simulink model "hexa_tilted_CAD_FxTESO_ANSFT"  (R2023a)
settings: Solver=ode4  StartTime=0.0  StopTime=60  FixedStep=0.01  RelTol=1e-3
model workspace (MAT data in the model file):
  hover_2m = [0  0  0  0  0  0; 0  0  0  0  0  0; 2  2  2  2  2  2; 0  0  0  0  0  0; 0  0  0  0  0  0; 0  0  0  0  0  0]
  square = [0  0  0  0  0  0; 0  0  0  0  0  0; 2.5  2.5  2.5  2.5  2.5  0; 0  0  0  0  0  0; 0  0  0  0  0  0; 0  0  0  0  0  0]
  tf = Simulink.Parameter
  tf.Value = 60
  tf.DataType = 'auto'
  tf.Complexity = 'real'
  tf.Dimensions = [1 1]
  tray0 = [0  0  0  0  0  0; 0  0  0  0  0  0; 0  5  5  5  5  0; 0  0  0  0  0  0; 0  0  0  0  0  0; 0  0  0  0  0  0]
  tray1 = [0  0  0  0  0  0; 0  0  0  0  0  0; 0  5  2.5  5  2.5  0; 0  0  0  0  0  0; 0  0  0  0  0  0; 0  0  0  0  0  0]
  tray2 = [0  2  2  -2  -2  0; 0  0  -2  -2  2  0; 0  5  2.5  5  2.5  0; 0  0  0  0  0  0; 0  0  0  0  0  0; 0  0  0  0  0  0]
  tray3 = [0  2  2  -2  -2  0; 0  0  -2  -2  2  0; 0  5  2.5  5  2.5  0; 0  0  0  0  0  0; 0  0  0  0  0  0; 0  0  0.785  1.57  0.785  0]
  tray4 = [0  2  2  -2  -2  0; 0  0  -2  -2  2  0; 0  5  2.5  5  2.5  0; 0  0.15  0.15  0.15  0.15  0; 0  0  0  0  0  0; 0  0  0.785  1.57  0.785  0]
  tray5 = [0  0  0  0  0  0; 0  0  0  0  0  0; 0  5  2.5  5  2.5  0; 0  0.15  0.15  0  0  0; 0  0  0.15  0.15  0  0; 0  0  0  0  0  0]
  tray_yaw = [0  0  0  0  0  0; 0  0  0  0  0  0; 0  5  2.5  5  2.5  0; 0  0  0  0  0  0; 0  0  0  0  0  0; 0  0  0.785  1.57  0.785  0]
undefined symbols (not defined in the file or in its folder): F, Light, MIL, smiData, X, Y, Z
libraries: sm_lib x229, nesl_utility x26, sharedtransform x2, robotcorelib x2, mspsensorlib x1, sensorinslib x1, simulink x1, aerolibwind2 x1, SignalEditorBlockLib x1
(part 1 of 6)
settings Model: Creator=adan  LastModifiedBy=adan
settings OptimizationCC: DefaultParameterBehavior=Inlined  EnhancedBackFolding=on  PassReuseOutputArgsAs=Individual arguments  ZeroExternalMemoryAtStartup=off  ZeroInternalMemoryAtStartup=off  OptimizeBlockOrder=speed  DifferentSizesBufferReuse=on  OptimizationCustomize=off  EfficientTunableParamExpr=on
settings DebuggingCC: ParameterTunabilityLossMsg=error
settings SFSimCC: MATLABDynamicMemAlloc=off
settings RTWCC: Description=Embedded Coder  SystemTargetFile=ert.tlc  TemplateMakefile=ert_default_tmf
settings CodeAppCC: ForceParamTrailComments=on  IgnoreCustomStorageClasses=off  OperatorAnnotations=on  SimulinkDataObjDesc=on  SFDataObjDesc=on  InsertBlockDesc=on
settings ERTTargetCC: TargetLangStandard=C99 (ISO)  GenerateSampleERTMain=on  InlinedParameterPlacement=NonHierarchical  ERTCustomFileTemplate=example_file_process.tlc

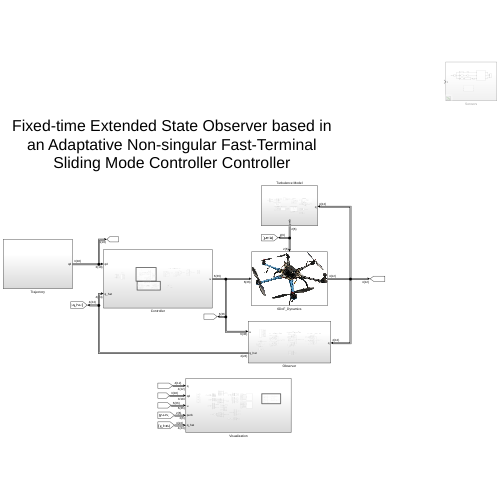
[thumbnail: Simulink's stored preview of the top-level diagram]
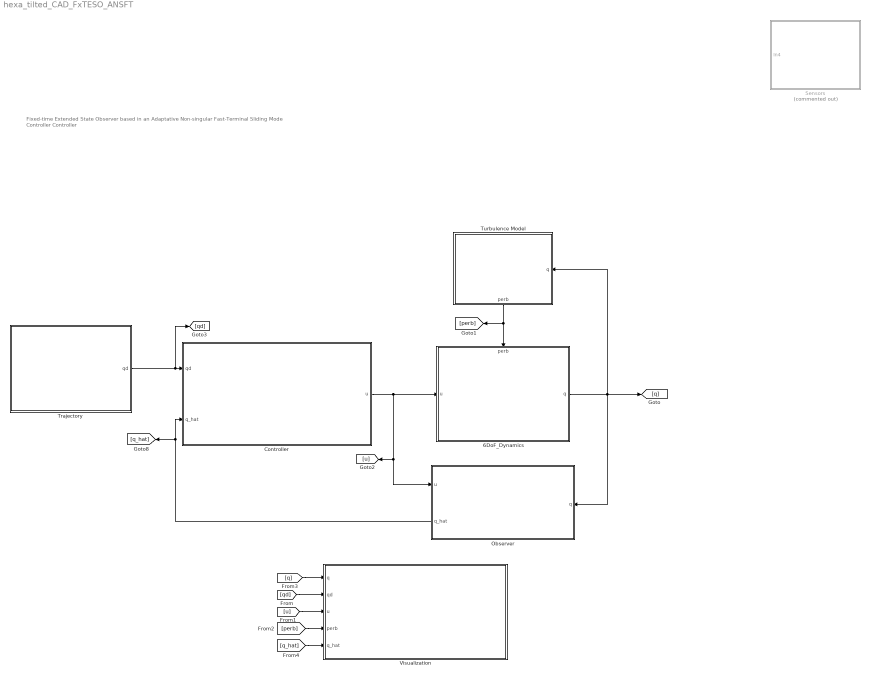
== system hexa_tilted_CAD_FxTESO_ANSFT ==
  note: Fixed-time Extended State Observer based in an Adaptative Non-singular Fast-Terminal Sliding Mode Controller Controller
  6DoF_Dynamics : Subsystem
      settings: PortSchema="{\"entries\":[{\"content\":{\"sides\":[{\"content\":{\"connectorIds\":[\"In1\"]},\"type\":\"ConnectorPlacement.EquallySpacedRectSide\",\"uuid\":\"d79ec49c-5563-41e0-ac59-6e897bc19fda\"},{\"content\":{\"connectorIds\":[\"Out1\"],\"side\":\"RIGHT\"},\"type\":\"ConnectorPlacement.EquallySpacedRectSide\",\"uuid\":\"1255043e-c90e-4bae-9fb4-4fa06f36f53e\"},{\"content\":{\"connectorIds\":[\"In2\"],\"side\":\"TOP\"},\"type\":\"ConnectorPlacement.EquallySpacedRectSide\",\"uuid\":\"823ada36-3f22-4ee3-87a1-180276f622bc\"}]},\"type\":\"ConnectorPlacement.EquallySpacedConnector\",\"uuid\":\"7403b609-b333-4977-a854-ed7a71f74338\"}],\"packageUris\":[\"http://schema.mathworks.com/mf0/Connector/R2020b\"],\"version\":\"1.0\"}"
      mask Display: image('/home/adan/Descargas/hexatilted.jpeg'); % Use "Edit Image" on toolstrip to change.
  Controller : Subsystem
  Observer : Subsystem
      settings: PortSchema="{\"entries\":[{\"content\":{\"sides\":[{\"content\":{\"connectorIds\":[\"In1\",\"Out1\"]},\"type\":\"ConnectorPlacement.EquallySpacedRectSide\",\"uuid\":\"d79ec49c-5563-41e0-ac59-6e897bc19fda\"},{\"content\":{\"connectorIds\":[\"In2\"],\"side\":\"RIGHT\"},\"type\":\"ConnectorPlacement.EquallySpacedRectSide\",\"uuid\":\"1255043e-c90e-4bae-9fb4-4fa06f36f53e\"},{\"content\":{\"side\":\"TOP\"},\"type\":\"ConnectorPlacement.EquallySpacedRectSide\",\"uuid\":\"823ada36-3f22-4ee3-87a1-180276f622bc\"}]},\"type\":\"ConnectorPlacement.EquallySpacedConnector\",\"uuid\":\"7403b609-b333-4977-a854-ed7a71f74338\"}],\"packageUris\":[\"http://schema.mathworks.com/mf0/Connector/R2020b\"],\"version\":\"1.0\"}"
  Sensors : Subsystem  Commented=on
  Trajectory : Subsystem
  Turbulence Model : Subsystem
      settings: PortSchema="{\"entries\":[{\"content\":{\"sides\":[{\"content\":{},\"type\":\"ConnectorPlacement.EquallySpacedRectSide\",\"uuid\":\"1a11629b-61d3-4a8e-8df8-8509e014e579\"},{\"content\":{\"connectorIds\":[\"In1\"],\"side\":\"RIGHT\"},\"type\":\"ConnectorPlacement.EquallySpacedRectSide\",\"uuid\":\"4b15c564-9714-4da5-9436-a08c0d95800f\"},{\"content\":{\"side\":\"TOP\"},\"type\":\"ConnectorPlacement.EquallySpacedRectSide\",\"uuid\":\"dd21b825-2def-4360-b27b-b8c6f475bfab\"},{\"content\":{\"connectorIds\":[\"Out1\"],\"side\":\"BOTTOM\"},\"type\":\"ConnectorPlacement.EquallySpacedRectSide\",\"uuid\":\"06c31a07-f778-4273-8a03-7a766e1c2883\"}]},\"type\":\"ConnectorPlacement.EquallySpacedConnector\",\"uuid\":\"4c6e67eb-825c-4dd0-a48b-2afa68ae74f5\"}],\"packageUris\":[\"http://schema.mathworks.com/mf0/Connector/R2020b\"],\"version\":\"1.0\"}"
  Visualization : Subsystem
  wires:
  Trajectory/1(qd) -> [qd], Controller/1(qd)
  Controller/1(u) -> 6DoF_Dynamics/1(u), [u], Observer/1(u)
  6DoF_Dynamics/1(q) -> Turbulence Model/1(q), [q], Observer/2(q)
  Observer/1(q_hat) -> [q_hat], Controller/2(q_hat)
  [qd] -> Visualization/2(qd)
  [u] -> Visualization/3(u)
  [perb] -> Visualization/4(perb)
  [q_hat] -> Visualization/5(q_hat)
  [q] -> Visualization/1(q)
  Turbulence Model/1(perb) -> 6DoF_Dynamics/2(perb), [perb]

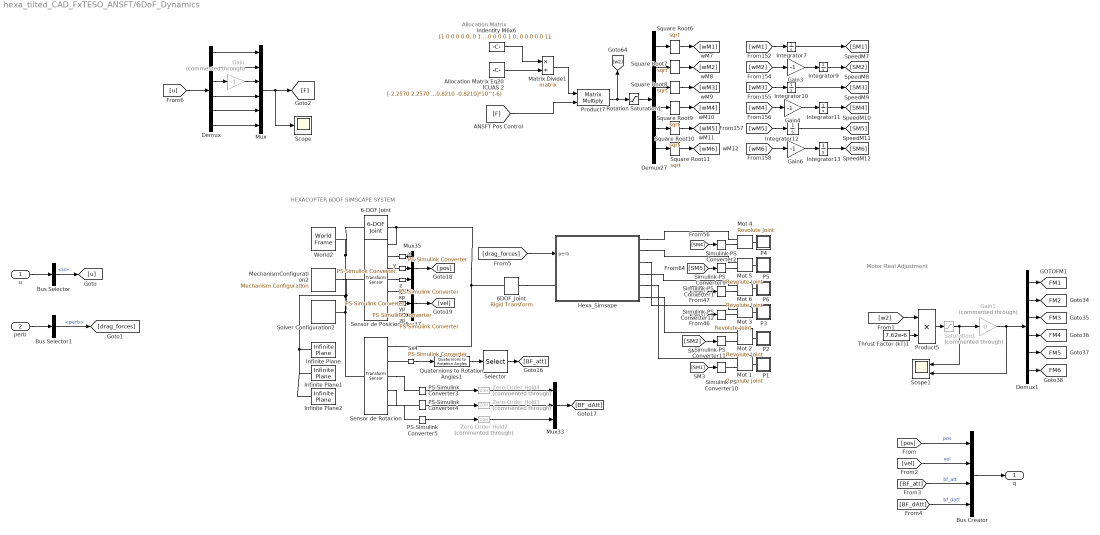
== system hexa_tilted_CAD_FxTESO_ANSFT/6DoF_Dynamics ==
  note: Motor Real Adjustment
  note: Allocation Matrix
  note: HEXACOPTER 6DOF SIMSCAPE SYSTEM
  u : Inport
  perb : Inport  Port=2
  6-DOF Joint : sm_lib/Joints/6-DOF Joint  JointMode=Normal  SenseConstraintForce=off  SenseConstraintForceX=off  SenseConstraintForceY=off  SenseConstraintForceZ=off  SenseConstraintTorque=off  SenseConstraintTorqueX=off  SenseConstraintTorqueY=off  SenseConstraintTorqueZ=off  SenseTotalForce=off  SenseTotalForceX=off  SenseTotalForceY=off  SenseTotalForceZ=off  SenseTotalTorque=off  SenseTotalTorqueX=off  SenseTotalTorqueY=off  SenseTotalTorqueZ=off  CompositeWrenchDir=FollowerOnBase  CompositeWrenchFrame=BaseFrame  PxEquilibriumPosition=0  PxEquilibriumPositionUnits=m  PxSpringStiffness=0  PxSpringStiffnessUnits=N/m  PxDampingCoefficient=0  PxDampingCoefficientUnits=N/(m/s)  PxTorqueActuationMode=NoTorque  PxMotionActuationMode=ComputedMotion  PxSensePosition=off  PxSenseVelocity=off  PxSenseAcceleration=off  PxSenseTorqueForce=off  PxSenseLowerLimitTorqueForce=off  PxSenseUpperLimitTorqueForce=off  PxLowerLimitSpecify=off  PxLowerLimitBound=-1  PxLowerLimitBoundUnits=m  PxLowerLimitStiffness=1e6  PxLowerLimitStiffnessUnits=N/m  PxLowerLimitDamping=1e3  PxLowerLimitDampingUnits=N/(m/s)  PxLowerLimitTransitionRegionWidth=1e-4  PxLowerLimitTransitionRegionWidthUnits=m  PxUpperLimitSpecify=off  PxUpperLimitBound=1  PxUpperLimitBoundUnits=m  PxUpperLimitStiffness=1e6  PxUpperLimitStiffnessUnits=N/m  PxUpperLimitDamping=1e3  PxUpperLimitDampingUnits=N/(m/s)  PxUpperLimitTransitionRegionWidth=1e-4  PxUpperLimitTransitionRegionWidthUnits=m  PxPositionTargetSpecify=off  PxPositionTargetPriority=High  PxPositionTargetValue=0  PxPositionTargetValueUnits=m  PxVelocityTargetSpecify=off  PxVelocityTargetPriority=High  PxVelocityTargetValue=0  PxVelocityTargetValueUnits=m/s  PyEquilibriumPosition=0  PyEquilibriumPositionUnits=m  PySpringStiffness=0  PySpringStiffnessUnits=N/m  PyDampingCoefficient=0  PyDampingCoefficientUnits=N/(m/s)  PyTorqueActuationMode=NoTorque  PyMotionActuationMode=ComputedMotion  PySensePosition=off  PySenseVelocity=off  PySenseAcceleration=off  PySenseTorqueForce=off  PySenseLowerLimitTorqueForce=off  PySenseUpperLimitTorqueForce=off  PyLowerLimitSpecify=off  PyLowerLimitBound=-1  PyLowerLimitBoundUnits=m  PyLowerLimitStiffness=1e6  PyLowerLimitStiffnessUnits=N/m  PyLowerLimitDamping=1e3  PyLowerLimitDampingUnits=N/(m/s)  PyLowerLimitTransitionRegionWidth=1e-4  PyLowerLimitTransitionRegionWidthUnits=m  PyUpperLimitSpecify=off  PyUpperLimitBound=1  PyUpperLimitBoundUnits=m  PyUpperLimitStiffness=1e6  PyUpperLimitStiffnessUnits=N/m  PyUpperLimitDamping=1e3  PyUpperLimitDampingUnits=N/(m/s)  PyUpperLimitTransitionRegionWidth=1e-4  PyUpperLimitTransitionRegionWidthUnits=m  PyPositionTargetSpecify=off  PyPositionTargetPriority=High  PyPositionTargetValue=0  PyPositionTargetValueUnits=m  PyVelocityTargetSpecify=off  PyVelocityTargetPriority=High  PyVelocityTargetValue=0  PyVelocityTargetValueUnits=m/s  PzEquilibriumPosition=0  PzEquilibriumPositionUnits=m  PzSpringStiffness=0  PzSpringStiffnessUnits=N/m  PzDampingCoefficient=0  PzDampingCoefficientUnits=N/(m/s)  PzTorqueActuationMode=NoTorque  PzMotionActuationMode=ComputedMotion  PzSensePosition=off  PzSenseVelocity=off  PzSenseAcceleration=off  PzSenseTorqueForce=off  PzSenseLowerLimitTorqueForce=off  PzSenseUpperLimitTorqueForce=off  PzLowerLimitSpecify=off  PzLowerLimitBound=-1  PzLowerLimitBoundUnits=m  PzLowerLimitStiffness=1e6  PzLowerLimitStiffnessUnits=N/m  PzLowerLimitDamping=1e3  PzLowerLimitDampingUnits=N/(m/s)  PzLowerLimitTransitionRegionWidth=1e-4  PzLowerLimitTransitionRegionWidthUnits=m  PzUpperLimitSpecify=off  PzUpperLimitBound=1  PzUpperLimitBoundUnits=m  PzUpperLimitStiffness=1e6  PzUpperLimitStiffnessUnits=N/m  PzUpperLimitDamping=1e3  PzUpperLimitDampingUnits=N/(m/s)  PzUpperLimitTransitionRegionWidth=1e-4  PzUpperLimitTransitionRegionWidthUnits=m  PzPositionTargetSpecify=on  PzPositionTargetPriority=High  PzPositionTargetValue=0.20  PzPositionTargetValueUnits=m  PzVelocityTargetSpecify=off  PzVelocityTargetPriority=High  PzVelocityTargetValue=0  PzVelocityTargetValueUnits=m/s  SphEqPosRotationMethod=None  SphEqPosRotationAngleUnits=deg  SphEqPosRotationStandardAxis=+Z  SphEqPosRotationAngle=0.0  SphEqPosRotationArbitraryAxis=[0 0 1]  SphEqPosFollAlignAxisA=+X  SphEqPosBaseAlignAxisA=+Y  SphEqPosFollAlignAxisB=+Y  SphEqPosBaseAlignAxisB=+Z  SphEqPosRotationSequenceAxes=FollowerAxes  SphEqPosRotationSequence=XYX  SphEqPosRotationSequenceAngles=[0 0 0]  SphEqPosRotationSequenceAnglesUnits=deg  SphEqPosRotationMatrix=[1 0 0; 0 1 0; 0 0 1]  SphEqPosQuaternion=[1 0 0 0]  SphSpringStiffness=0  SphSpringStiffnessUnits=N*m/deg  SphDampingCoefficient=0  SphDampingCoefficientUnits=N*m/(deg/s)  SphActuateTorqueX=off  SphActuateTorqueY=off  SphActuateTorqueZ=off  SphActuateTorque=off  SphTorqueActuationMode=NoTorque  SphMotionActuationMode=ComputedMotion  SphActuationFrame=BaseFrame  SphSensePosition=off  SphSenseVelocityX=off  SphSenseVelocityY=off  SphSenseVelocityZ=off  SphSenseVelocity=off  SphSenseAccelerationX=off  SphSenseAccelerationY=off  SphSenseAccelerationZ=off  SphSenseAcceleration=off  SphSenseTorqueX=off  SphSenseTorqueY=off  SphSenseTorqueZ=off  SphSenseTorqueForce=off  SphSenseLowerLimitTorqueMag=off  SphSenseUpperLimitTorqueMag=off  SphSensingFrame=BaseFrame  SphLowerLimitSpecify=off  SphLowerLimitBound=15  SphLowerLimitBoundUnits=deg  SphLowerLimitStiffness=1e4  SphLowerLimitStiffnessUnits=N*m/deg  SphLowerLimitDamping=10  SphLowerLimitDampingUnits=N*m/(deg/s)  SphLowerLimitTransitionRegionWidth=0.1  SphLowerLimitTransitionRegionWidthUnits=deg  SphUpperLimitSpecify=off  SphUpperLimitBound=45  SphUpperLimitBoundUnits=deg  SphUpperLimitStiffness=1e4  SphUpperLimitStiffnessUnits=N*m/deg  SphUpperLimitDamping=10  SphUpperLimitDampingUnits=N*m/(deg/s)  SphUpperLimitTransitionRegionWidth=0.1  SphUpperLimitTransitionRegionWidthUnits=deg  SphPositionTargetRotationMethod=StandardAxis  SphPositionTargetRotationAngleUnits=deg  SphPositionTargetRotationStandardAxis=+Z  SphPositionTargetRotationAngle=-45  SphPositionTargetRotationArbitraryAxis=[0 0 1]  SphPositionTargetFollAlignAxisA=+X  SphPositionTargetBaseAlignAxisA=+Y  SphPositionTargetFollAlignAxisB=+Y  SphPositionTargetBaseAlignAxisB=+Z  SphPositionTargetRotationSequenceAxes=FollowerAxes  SphPositionTargetRotationSequence=XYX  SphPositionTargetRotationSequenceAngles=[0 0 0]  SphPositionTargetRotationSequenceAnglesUnits=deg  SphPositionTargetRotationMatrix=[1 0 0; 0 1 0; 0 0 1]  SphPositionTargetQuaternion=[1 0 0 0]  SphPositionTargetSpecify=off  SphPositionTargetPriority=High  SphVelocityTargetValue=[0 0 0]  SphVelocityTargetValueUnits=deg/s  SphVelocityTargetSpecify=off  SphVelocityTargetPriority=High  SphVelocityTargetInFollowerFrame=on
  6DOF_Joint : sm_lib/Frames and Transforms/Rigid Transform  TranslationMethod=Cartesian  TranslationStandardOffset=-0.185  TranslationStandardOffsetUnits=m  TranslationStandardAxis=+Z  TranslationCartesianOffset=[0.0195 0.01 -0.26]  TranslationCartesianOffsetUnits=m  TranslationROffset=0  TranslationROffsetUnits=m  TranslationZOffset=0  TranslationZOffsetUnits=m  TranslationThetaOffset=0  TranslationThetaOffsetUnits=deg  RotationMethod=RotationMatrix  RotationAngleUnits=deg  RotationStandardAxis=+Z  RotationAngle=0.0  RotationArbitraryAxis=[0 0 1]  FollAlignAxisA=+X  BaseAlignAxisA=+Y  FollAlignAxisB=+Y  BaseAlignAxisB=+Z  RotationSequenceAxes=FollowerAxes  RotationSequence=XYX  RotationSequenceAngles=[0 0 0]  RotationSequenceAnglesUnits=deg  RotationMatrix=[1 0 0; 0 1 0; 0 0 1]  Quaternion=[1 0 0 0]
  Allocation Matrix Eq20 ICUAS 2 : Constant  Value=[-2.2570 2.2570 0 -2.2570 2.2570 0; 1.3030 1.3030 -2.6060 1.3030 1.3030 -2.6060; 7.160 7.160 7.160 7.160 7.160 7.160; 1.6370 1.6370 0 -1.6370 -1.6370 0; -0.945 0.945 1.891 0.945 -0.945 -1.891; 0.8210 -0.8210 0.8210 -0.8210 0.8210 -0.8210]*10^(-6)
  Bus Creator : BusCreator  Inputs=4
  Bus Selector : BusSelector  OutputSignals=u
  Bus Selector1 : BusSelector  OutputSignals=perb
  Demux : Demux  Outputs=6
  Demux1 : Demux  Outputs=6
  Demux27 : Demux  Outputs=6
  Gain : Gain  Commented=through  Gain=-1
  Gain1 : Gain  Commented=through  Gain=0
  Gain3 : Gain  Gain=-1
  Gain4 : Gain  Gain=-1
  Gain6 : Gain  Gain=-1
  Hexa_Simsape : Subsystem
      mask Display: image('$imagefile'); % Use "Edit Image" on toolstrip to change.
  Indentity M6x6 : Constant  Value=[1 0 0 0 0 0; 0 1 0 0 0 0; 0 0 1 0 0 0; 0 0 0 1 0 0; 0 0 0 0 1 0; 0 0 0 0 0 1];
  Infinite Plane : sm_lib/Curves and Surfaces/Infinite Plane  GraphicType=Rectangle  GraphicPlaneWidth=8  GraphicPlaneWidthUnits=m  GraphicPlaneHeight=5  GraphicPlaneHeightUnits=m  GraphicVisPropType=SimpleVisualProperties  GraphicDiffuseColor=[1 1 0.06667]  GraphicOpacity=0.25  GraphicSpecularColor=[1 1 1]  GraphicAmbientColor=[1 1 1]  GraphicEmissiveColor=[1 1 1]  GraphicShininess=75
  Infinite Plane1 : sm_lib/Curves and Surfaces/Infinite Plane  GraphicType=Rectangle  GraphicPlaneWidth=8  GraphicPlaneWidthUnits=m  GraphicPlaneHeight=0.01  GraphicPlaneHeightUnits=m  GraphicVisPropType=SimpleVisualProperties  GraphicDiffuseColor=[1 1 0.06667]  GraphicOpacity=0.5  GraphicSpecularColor=[0.5 0.5 0.5 1.0]  GraphicAmbientColor=[0.15 0.15 0.15 1.0]  GraphicEmissiveColor=[0.0 0.0 0.0 1.0]  GraphicShininess=75
  Infinite Plane2 : sm_lib/Curves and Surfaces/Infinite Plane  GraphicType=Rectangle  GraphicPlaneWidth=0.01  GraphicPlaneWidthUnits=m  GraphicPlaneHeight=5  GraphicPlaneHeightUnits=m  GraphicVisPropType=SimpleVisualProperties  GraphicDiffuseColor=[1 1 0.06667]  GraphicOpacity=0.5  GraphicSpecularColor=[0.5 0.5 0.5 1.0]  GraphicAmbientColor=[0.15 0.15 0.15 1.0]  GraphicEmissiveColor=[0.0 0.0 0.0 1.0]  GraphicShininess=75
  Integrator{7,9..13} (6 alike) : Integrator
  Matrix Divide1 : Product  Inputs=*/  Multiplication=Matrix(*)
  MechanismConfiguration2 : sm_lib/Utilities/Mechanism Configuration  UniformGravity=Constant  GravityVector=[0 0 -9.80665]  GravityVectorUnits=m/s^2  LinearizationDelta=0.01  JointModeTransitionNonlinearIterations=2
  Mot 1 : sm_lib/Joints/Revolute Joint  JointMode=Normal  SenseConstraintForce=off  SenseConstraintForceX=off  SenseConstraintForceY=off  SenseConstraintForceZ=off  SenseConstraintTorque=off  SenseConstraintTorqueX=off  SenseConstraintTorqueY=off  SenseConstraintTorqueZ=off  SenseTotalForce=off  SenseTotalForceX=off  SenseTotalForceY=off  SenseTotalForceZ=off  SenseTotalTorque=off  SenseTotalTorqueX=off  SenseTotalTorqueY=off  SenseTotalTorqueZ=off  CompositeWrenchDir=FollowerOnBase  CompositeWrenchFrame=BaseFrame  EquilibriumPosition=0  EquilibriumPositionUnits=deg  SpringStiffness=0  SpringStiffnessUnits=N*m/deg  DampingCoefficient=0  DampingCoefficientUnits=N*m/(deg/s)  TorqueActuationMode=ComputedTorque  MotionActuationMode=InputMotion  SensePosition=off  SenseVelocity=off  SenseAcceleration=off  SenseTorqueForce=off  SenseLowerLimitTorqueForce=off  SenseUpperLimitTorqueForce=off  LowerLimitSpecify=off  LowerLimitBound=-90  LowerLimitBoundUnits=deg  LowerLimitStiffness=1e4  LowerLimitStiffnessUnits=N*m/deg  LowerLimitDamping=10  LowerLimitDampingUnits=N*m/(deg/s)  LowerLimitTransitionRegionWidth=0.1  LowerLimitTransitionRegionWidthUnits=deg  UpperLimitSpecify=off  UpperLimitBound=90  UpperLimitBoundUnits=deg  UpperLimitStiffness=1e4  UpperLimitStiffnessUnits=N*m/deg  UpperLimitDamping=10  UpperLimitDampingUnits=N*m/(deg/s)  UpperLimitTransitionRegionWidth=0.1  UpperLimitTransitionRegionWidthUnits=deg  PositionTargetSpecify=on  PositionTargetPriority=Low  PositionTargetValue=smiData.RevoluteJoint(1).Rz.Pos  PositionTargetValueUnits=deg  VelocityTargetSpecify=off  VelocityTargetPriority=High  VelocityTargetValue=0  VelocityTargetValueUnits=deg/s
  Mot 2 : sm_lib/Joints/Revolute Joint  JointMode=Normal  SenseConstraintForce=off  SenseConstraintForceX=off  SenseConstraintForceY=off  SenseConstraintForceZ=off  SenseConstraintTorque=off  SenseConstraintTorqueX=off  SenseConstraintTorqueY=off  SenseConstraintTorqueZ=off  SenseTotalForce=off  SenseTotalForceX=off  SenseTotalForceY=off  SenseTotalForceZ=off  SenseTotalTorque=off  SenseTotalTorqueX=off  SenseTotalTorqueY=off  SenseTotalTorqueZ=off  CompositeWrenchDir=FollowerOnBase  CompositeWrenchFrame=BaseFrame  EquilibriumPosition=0  EquilibriumPositionUnits=deg  SpringStiffness=0  SpringStiffnessUnits=N*m/deg  DampingCoefficient=0  DampingCoefficientUnits=N*m/(deg/s)  TorqueActuationMode=ComputedTorque  MotionActuationMode=InputMotion  SensePosition=off  SenseVelocity=off  SenseAcceleration=off  SenseTorqueForce=off  SenseLowerLimitTorqueForce=off  SenseUpperLimitTorqueForce=off  LowerLimitSpecify=off  LowerLimitBound=-90  LowerLimitBoundUnits=deg  LowerLimitStiffness=1e4  LowerLimitStiffnessUnits=N*m/deg  LowerLimitDamping=10  LowerLimitDampingUnits=N*m/(deg/s)  LowerLimitTransitionRegionWidth=0.1  LowerLimitTransitionRegionWidthUnits=deg  UpperLimitSpecify=off  UpperLimitBound=90  UpperLimitBoundUnits=deg  UpperLimitStiffness=1e4  UpperLimitStiffnessUnits=N*m/deg  UpperLimitDamping=10  UpperLimitDampingUnits=N*m/(deg/s)  UpperLimitTransitionRegionWidth=0.1  UpperLimitTransitionRegionWidthUnits=deg  PositionTargetSpecify=on  PositionTargetPriority=Low  PositionTargetValue=smiData.RevoluteJoint(2).Rz.Pos  PositionTargetValueUnits=deg  VelocityTargetSpecify=off  VelocityTargetPriority=High  VelocityTargetValue=0  VelocityTargetValueUnits=deg/s
  Mot 3 : sm_lib/Joints/Revolute Joint  JointMode=Normal  SenseConstraintForce=off  SenseConstraintForceX=off  SenseConstraintForceY=off  SenseConstraintForceZ=off  SenseConstraintTorque=off  SenseConstraintTorqueX=off  SenseConstraintTorqueY=off  SenseConstraintTorqueZ=off  SenseTotalForce=off  SenseTotalForceX=off  SenseTotalForceY=off  SenseTotalForceZ=off  SenseTotalTorque=off  SenseTotalTorqueX=off  SenseTotalTorqueY=off  SenseTotalTorqueZ=off  CompositeWrenchDir=FollowerOnBase  CompositeWrenchFrame=BaseFrame  EquilibriumPosition=0  EquilibriumPositionUnits=deg  SpringStiffness=0  SpringStiffnessUnits=N*m/deg  DampingCoefficient=0  DampingCoefficientUnits=N*m/(deg/s)  TorqueActuationMode=ComputedTorque  MotionActuationMode=InputMotion  SensePosition=off  SenseVelocity=off  SenseAcceleration=off  SenseTorqueForce=off  SenseLowerLimitTorqueForce=off  SenseUpperLimitTorqueForce=off  LowerLimitSpecify=off  LowerLimitBound=-90  LowerLimitBoundUnits=deg  LowerLimitStiffness=1e4  LowerLimitStiffnessUnits=N*m/deg  LowerLimitDamping=10  LowerLimitDampingUnits=N*m/(deg/s)  LowerLimitTransitionRegionWidth=0.1  LowerLimitTransitionRegionWidthUnits=deg  UpperLimitSpecify=off  UpperLimitBound=90  UpperLimitBoundUnits=deg  UpperLimitStiffness=1e4  UpperLimitStiffnessUnits=N*m/deg  UpperLimitDamping=10  UpperLimitDampingUnits=N*m/(deg/s)  UpperLimitTransitionRegionWidth=0.1  UpperLimitTransitionRegionWidthUnits=deg  PositionTargetSpecify=on  PositionTargetPriority=Low  PositionTargetValue=smiData.RevoluteJoint(3).Rz.Pos  PositionTargetValueUnits=deg  VelocityTargetSpecify=off  VelocityTargetPriority=High  VelocityTargetValue=0  VelocityTargetValueUnits=deg/s
  Mot 4 : sm_lib/Joints/Revolute Joint  JointMode=Normal  SenseConstraintForce=off  SenseConstraintForceX=off  SenseConstraintForceY=off  SenseConstraintForceZ=off  SenseConstraintTorque=off  SenseConstraintTorqueX=off  SenseConstraintTorqueY=off  SenseConstraintTorqueZ=off  SenseTotalForce=off  SenseTotalForceX=off  SenseTotalForceY=off  SenseTotalForceZ=off  SenseTotalTorque=off  SenseTotalTorqueX=off  SenseTotalTorqueY=off  SenseTotalTorqueZ=off  CompositeWrenchDir=FollowerOnBase  CompositeWrenchFrame=BaseFrame  EquilibriumPosition=0  EquilibriumPositionUnits=deg  SpringStiffness=0  SpringStiffnessUnits=N*m/deg  DampingCoefficient=0  DampingCoefficientUnits=N*m/(deg/s)  TorqueActuationMode=ComputedTorque  MotionActuationMode=InputMotion  SensePosition=off  SenseVelocity=off  SenseAcceleration=off  SenseTorqueForce=off  SenseLowerLimitTorqueForce=off  SenseUpperLimitTorqueForce=off  LowerLimitSpecify=off  LowerLimitBound=-90  LowerLimitBoundUnits=deg  LowerLimitStiffness=1e4  LowerLimitStiffnessUnits=N*m/deg  LowerLimitDamping=10  LowerLimitDampingUnits=N*m/(deg/s)  LowerLimitTransitionRegionWidth=0.1  LowerLimitTransitionRegionWidthUnits=deg  UpperLimitSpecify=off  UpperLimitBound=90  UpperLimitBoundUnits=deg  UpperLimitStiffness=1e4  UpperLimitStiffnessUnits=N*m/deg  UpperLimitDamping=10  UpperLimitDampingUnits=N*m/(deg/s)  UpperLimitTransitionRegionWidth=0.1  UpperLimitTransitionRegionWidthUnits=deg  PositionTargetSpecify=on  PositionTargetPriority=Low  PositionTargetValue=smiData.RevoluteJoint(5).Rz.Pos  PositionTargetValueUnits=deg  VelocityTargetSpecify=off  VelocityTargetPriority=High  VelocityTargetValue=0  VelocityTargetValueUnits=deg/s
  Mot 5 : sm_lib/Joints/Revolute Joint  JointMode=Normal  SenseConstraintForce=off  SenseConstraintForceX=off  SenseConstraintForceY=off  SenseConstraintForceZ=off  SenseConstraintTorque=off  SenseConstraintTorqueX=off  SenseConstraintTorqueY=off  SenseConstraintTorqueZ=off  SenseTotalForce=off  SenseTotalForceX=off  SenseTotalForceY=off  SenseTotalForceZ=off  SenseTotalTorque=off  SenseTotalTorqueX=off  SenseTotalTorqueY=off  SenseTotalTorqueZ=off  CompositeWrenchDir=FollowerOnBase  CompositeWrenchFrame=BaseFrame  EquilibriumPosition=0  EquilibriumPositionUnits=deg  SpringStiffness=0  SpringStiffnessUnits=N*m/deg  DampingCoefficient=0  DampingCoefficientUnits=N*m/(deg/s)  TorqueActuationMode=ComputedTorque  MotionActuationMode=InputMotion  SensePosition=off  SenseVelocity=off  SenseAcceleration=off  SenseTorqueForce=off  SenseLowerLimitTorqueForce=off  SenseUpperLimitTorqueForce=off  LowerLimitSpecify=off  LowerLimitBound=-90  LowerLimitBoundUnits=deg  LowerLimitStiffness=1e4  LowerLimitStiffnessUnits=N*m/deg  LowerLimitDamping=10  LowerLimitDampingUnits=N*m/(deg/s)  LowerLimitTransitionRegionWidth=0.1  LowerLimitTransitionRegionWidthUnits=deg  UpperLimitSpecify=off  UpperLimitBound=90  UpperLimitBoundUnits=deg  UpperLimitStiffness=1e4  UpperLimitStiffnessUnits=N*m/deg  UpperLimitDamping=10  UpperLimitDampingUnits=N*m/(deg/s)  UpperLimitTransitionRegionWidth=0.1  UpperLimitTransitionRegionWidthUnits=deg  PositionTargetSpecify=on  PositionTargetPriority=Low  PositionTargetValue=smiData.RevoluteJoint(6).Rz.Pos  PositionTargetValueUnits=deg  VelocityTargetSpecify=off  VelocityTargetPriority=High  VelocityTargetValue=0  VelocityTargetValueUnits=deg/s
  Mot 6 : sm_lib/Joints/Revolute Joint  JointMode=Normal  SenseConstraintForce=off  SenseConstraintForceX=off  SenseConstraintForceY=off  SenseConstraintForceZ=off  SenseConstraintTorque=off  SenseConstraintTorqueX=off  SenseConstraintTorqueY=off  SenseConstraintTorqueZ=off  SenseTotalForce=off  SenseTotalForceX=off  SenseTotalForceY=off  SenseTotalForceZ=off  SenseTotalTorque=off  SenseTotalTorqueX=off  SenseTotalTorqueY=off  SenseTotalTorqueZ=off  CompositeWrenchDir=FollowerOnBase  CompositeWrenchFrame=BaseFrame  EquilibriumPosition=0  EquilibriumPositionUnits=deg  SpringStiffness=0  SpringStiffnessUnits=N*m/deg  DampingCoefficient=0  DampingCoefficientUnits=N*m/(deg/s)  TorqueActuationMode=ComputedTorque  MotionActuationMode=InputMotion  SensePosition=off  SenseVelocity=off  SenseAcceleration=off  SenseTorqueForce=off  SenseLowerLimitTorqueForce=off  SenseUpperLimitTorqueForce=off  LowerLimitSpecify=off  LowerLimitBound=-90  LowerLimitBoundUnits=deg  LowerLimitStiffness=1e4  LowerLimitStiffnessUnits=N*m/deg  LowerLimitDamping=10  LowerLimitDampingUnits=N*m/(deg/s)  LowerLimitTransitionRegionWidth=0.1  LowerLimitTransitionRegionWidthUnits=deg  UpperLimitSpecify=off  UpperLimitBound=90  UpperLimitBoundUnits=deg  UpperLimitStiffness=1e4  UpperLimitStiffnessUnits=N*m/deg  UpperLimitDamping=10  UpperLimitDampingUnits=N*m/(deg/s)  UpperLimitTransitionRegionWidth=0.1  UpperLimitTransitionRegionWidthUnits=deg  PositionTargetSpecify=on  PositionTargetPriority=Low  PositionTargetValue=smiData.RevoluteJoint(4).Rz.Pos  PositionTargetValueUnits=deg  VelocityTargetSpecify=off  VelocityTargetPriority=High  VelocityTargetValue=0  VelocityTargetValueUnits=deg/s
  Mux : Mux  Inputs=6
  Mux33 : Mux  Inputs=3
  Mux35 : Mux  Inputs=3
  Mux37 : Mux  Inputs=3
  P1 : Subsystem
  P2 : Subsystem
  P3 : Subsystem
  P4 : Subsystem
  P5 : Subsystem
  P6 : Subsystem
  PS-Simulink Converter3 : nesl_utility/PS-Simulink Converter  PhysicalDomain=network_engine_domain  SubClassName=ps_output  LeftPortType=input  RightPortType=output  PseudoPeriodic=off  Frequencies=[]  VectorFormat=1-D array  Unit=inherit  AffineConversion=off
  PS-Simulink Converter4 : nesl_utility/PS-Simulink Converter  PhysicalDomain=network_engine_domain  SubClassName=ps_output  LeftPortType=input  RightPortType=output  PseudoPeriodic=off  Frequencies=[]  VectorFormat=1-D array  Unit=inherit  AffineConversion=off
  PS-Simulink Converter5 : nesl_utility/PS-Simulink Converter  PhysicalDomain=network_engine_domain  SubClassName=ps_output  LeftPortType=input  RightPortType=output  PseudoPeriodic=off  Frequencies=[]  VectorFormat=1-D array  Unit=inherit  AffineConversion=off
  Product5 : Product
  Product7 : Product  Multiplication=Matrix(*)
  Quaternions to Rotation Angles1 : sharedtransform/Quaternions to Rotation Angles  rotationOrder=ZYX  aMode=aMode
  Rotation Saturation1 : Saturate  UpperLimit=1.4e6  LowerLimit=0
  Saturation1 : Saturate  Commented=through  UpperLimit=10  LowerLimit=0
  Scope : Scope
  Scope1 : Scope  NumInputPorts=2
  Selector : Selector  InputPortWidth=3  IndexOptions=Index vector (dialog)  Indices=[3 2 1]  OutputSizes=1
  Sensor de Posicion : sm_lib/Frames and Transforms/Transform Sensor  MeasurementFrame=World  RotationSequence=XYX  SenseAngle=off  SenseAxis=off  SenseQ=off  SenseR=off  SenseRotationSequence=off  SenseOmegaX=off  SenseOmegaY=off  SenseOmegaZ=off  SenseQDot=off  SenseRDot=off  SenseRotationSequenceDot=off  SenseAlphaX=off  SenseAlphaY=off  SenseAlphaZ=off  SenseQDDot=off  SenseRDDot=off  SenseX=on  SenseY=on  SenseZ=on  SenseRad=off  SenseAzim=off  SenseDist=off  SenseInc=off  SenseXDot=on  SenseYDot=on  SenseZDot=on  SenseRadDot=off  SenseAzimDot=off  SenseDistDot=off  SenseIncDot=off  SenseXDDot=off  SenseYDDot=off  SenseZDDot=off  SenseRadDDot=off  SenseAzimDDot=off  SenseDistDDot=off  SenseIncDDot=off
  Sensor de Rotacion : sm_lib/Frames and Transforms/Transform Sensor  MeasurementFrame=Follower  RotationSequence=XYX  SenseAngle=off  SenseAxis=off  SenseQ=on  SenseR=off  SenseRotationSequence=off  SenseOmegaX=on  SenseOmegaY=on  SenseOmegaZ=on  SenseQDot=off  SenseRDot=off  SenseRotationSequenceDot=off  SenseAlphaX=off  SenseAlphaY=off  SenseAlphaZ=off  SenseQDDot=off  SenseRDDot=off  SenseX=off  SenseY=off  SenseZ=off  SenseRad=off  SenseAzim=off  SenseDist=off  SenseInc=off  SenseXDot=off  SenseYDot=off  SenseZDot=off  SenseRadDot=off  SenseAzimDot=off  SenseDistDot=off  SenseIncDot=off  SenseXDDot=off  SenseYDDot=off  SenseZDDot=off  SenseRadDDot=off  SenseAzimDDot=off  SenseDistDDot=off  SenseIncDDot=off
  Simulink-PS Converter{1..2,9..12} (6 alike) : nesl_utility/Simulink-PS Converter  PhysicalDomain=network_engine_domain  SubClassName=ps_input  LeftPortType=input  RightPortType=output  PseudoPeriodic=off  Frequencies=[]  NoiseDistribution=none  NoiseParameters=[]  Unit=rad  AffineConversion=off  FilteringAndDerivatives=filter  SimscapeFilterOrder=2  InputFilterTimeConstant=0.01  UdotUserProvided=0
  Solver Configuration2 : nesl_utility/Solver Configuration  PhysicalDomain=network_engine_domain  SubClassName=solver  LeftPortType=input  RightPortType=generic  Tones=[]  Harmonics=[]  SimulateNoise=off  Profile=off  UseLocalSampling=off  EnableSwitchedLinearOptims=on  FrequencyDomain=off  UseCCode=off  RelTol=0.001  AbsTol=1e-06  MinStep=1e-09  ToWorkspace=off  RevertToSquareIcSolve=off  NumHomotopyIterations=100  PhasorMode=off  PhasorModeNumHarmonics=1  ConsistencySolver=NEWTON_FTOL  IndexReductionMethod=DerivativeReplacement  DoDC=off  ResidualTolerance=1e-09  ConsistencyTolSource=GLOBAL  ConsistencyAbsTol=0.001  ConsistencyRelTol=0.001  ConsistencyTolFactor=0.001  UseLocalSolver=off  LocalSolverChoice=NE_BACKWARD_EULER_ADVANCER  ResolveIndetEquations=on  FunctionEvalNumThread=1  LocalSolverSampleTime=0.01  DoFixedCost=off  MaxNonlinIter=3  MaxModeIter=2  ComputeImpulses=off  ImpulseIterations=2  LinearAlgebra=Full  LinearAlgebraNumThread=0  EquationFormulation=NE_TIME_EF  DelaysMemoryBudget=1024  AutomaticFiltering=on  FilteringTimeConstant=0.001  PartitionStorageMethod=AS_NEEDED  PartitionMemoryBudget=1024  PartitionMethod=ROBUST
  Square Root{6..11} (6 alike) : Sqrt
  Sx4 : nesl_utility/PS-Simulink Converter  PhysicalDomain=network_engine_domain  SubClassName=ps_output  LeftPortType=input  RightPortType=output  PseudoPeriodic=off  Frequencies=[]  VectorFormat=1-D array  Unit=inherit  AffineConversion=on
  Thrust Factor (kT)1 : Constant  Value=7.62e-6
  World2 : sm_lib/Frames and Transforms/World Frame
  Zero-Order Hold2 : ZeroOrderHold  Commented=through  SampleTime=-1
  Zero-Order Hold3 : ZeroOrderHold  Commented=through  SampleTime=-1
  Zero-Order Hold4 : ZeroOrderHold  Commented=through  SampleTime=-1
  x : nesl_utility/PS-Simulink Converter  PhysicalDomain=network_engine_domain  SubClassName=ps_output  LeftPortType=input  RightPortType=output  PseudoPeriodic=off  Frequencies=[]  VectorFormat=1-D array  Unit=inherit  AffineConversion=on
  xp : nesl_utility/PS-Simulink Converter  PhysicalDomain=network_engine_domain  SubClassName=ps_output  LeftPortType=input  RightPortType=output  PseudoPeriodic=off  Frequencies=[]  VectorFormat=1-D array  Unit=inherit  AffineConversion=on
  y : nesl_utility/PS-Simulink Converter  PhysicalDomain=network_engine_domain  SubClassName=ps_output  LeftPortType=input  RightPortType=output  PseudoPeriodic=off  Frequencies=[]  VectorFormat=1-D array  Unit=inherit  AffineConversion=on
  yp : nesl_utility/PS-Simulink Converter  PhysicalDomain=network_engine_domain  SubClassName=ps_output  LeftPortType=input  RightPortType=output  PseudoPeriodic=off  Frequencies=[]  VectorFormat=1-D array  Unit=inherit  AffineConversion=on
  z : nesl_utility/PS-Simulink Converter  PhysicalDomain=network_engine_domain  SubClassName=ps_output  LeftPortType=input  RightPortType=output  PseudoPeriodic=off  Frequencies=[]  VectorFormat=1-D array  Unit=inherit  AffineConversion=on
  zp : nesl_utility/PS-Simulink Converter  PhysicalDomain=network_engine_domain  SubClassName=ps_output  LeftPortType=input  RightPortType=output  PseudoPeriodic=off  Frequencies=[]  VectorFormat=1-D array  Unit=inherit  AffineConversion=on
  q : Outport
  tag scope: FM1=global, FM2=global, FM3=global, FM4=global, FM5=global, FM6=global
  wires:
  Demux1/3 -> [FM3]
  Integrator13/1 -> [SM6]
  [w2] -> Product5/1
  Thrust Factor (kT)1/1 -> Product5/2
  Square Root8/1 -> [wM3]
  Square Root7/1 -> [wM2]
  [wM6] -> Gain6/1
  [wM1] -> Integrator7/1
  Square Root6/1 -> [wM1]
  Integrator11/1 -> [SM4]
  Demux27/4 -> Square Root9/1
  Demux1/5 -> [FM5]
  [wM3] -> Integrator10/1
  Integrator9/1 -> [SM2]
  Indentity M6x6/1 -> Matrix Divide1/1
  Quaternions to Rotation Angles1/1 -> Selector/1
  Demux27/2 -> Square Root7/1
  PS-Simulink Converter4/1 -> Zero-Order Hold3/1
  Allocation Matrix Eq20 ICUAS 2/1 -> Matrix Divide1/2
  Gain3/1 -> Integrator9/1
  Integrator7/1 -> [SM1]
  Integrator12/1 -> [SM5]
  z/1 -> Mux35/3
  Square Root10/1 -> [wM5]
  yp/1 -> Mux37/2
  Product7/1 -> Rotation Saturation1/1, [w2]
  [SM4] -> Simulink-PS Converter2/1
  Rotation Saturation1/1 -> Demux27/1
  Demux1/1 -> [FM1]
  Gain6/1 -> Integrator13/1
  Integrator10/1 -> [SM3]
  Demux27/6 -> Square Root11/1
  [SM3] -> Simulink-PS Converter12/1
  x/1 -> Mux35/1
  [SM5] -> Simulink-PS Converter9/1
  Mux33/1 -> [BF_dAtt]
  Saturation1/1 -> Scope1/1, Gain1/1
  Zero-Order Hold4/1 -> Mux33/1
  Demux1/2 -> [FM2]
  Gain4/1 -> Integrator11/1
  Square Root9/1 -> [wM4]
  [SM2] -> Simulink-PS Converter11/1
  Square Root11/1 -> [wM6]
  [F] -> Product7/2
  Mux37/1 -> [vel]
  Sx4/1 -> Quaternions to Rotation Angles1/1
  Demux1/4 -> [FM4]
  Demux27/3 -> Square Root8/1
  Mux35/1 -> [pos]
  zp/1 -> Mux37/3
  Demux1/6 -> [FM6]
  [SM6] -> Simulink-PS Converter1/1
  Demux27/1 -> Square Root6/1
  Product5/1 -> Saturation1/1
  xp/1 -> Mux37/1
  Demux27/5 -> Square Root10/1
  [wM2] -> Gain3/1
  [wM5] -> Integrator12/1
  Zero-Order Hold2/1 -> Mux33/3
  [wM4] -> Gain4/1
  Zero-Order Hold3/1 -> Mux33/2
  PS-Simulink Converter5/1 -> Zero-Order Hold2/1
  y/1 -> Mux35/2
  [SM1] -> Simulink-PS Converter10/1
  PS-Simulink Converter3/1 -> Zero-Order Hold4/1
  Matrix Divide1/1 -> Product7/1
  u/1 -> Bus Selector/1
  Bus Selector/1 -> [u]  "<u>"
  [pos] -> Bus Creator/1  "pos"
  [vel] -> Bus Creator/2  "vel"
  [BF_att] -> Bus Creator/3  "bf_att"
  [BF_dAtt] -> Bus Creator/4  "bf_datt"
  Bus Creator/1 -> q/1
  perb/1 -> Bus Selector1/1
  Bus Selector1/1 -> [drag_forces]  "<perb>"
  [drag_forces] -> Hexa_Simsape/1(perb)
  [u] -> Demux/1
  Demux/1 -> Mux/1
  Demux/2 -> Mux/2
  Demux/3 -> Gain/1
  Demux/4 -> Mux/4
  Demux/5 -> Mux/5
  Demux/6 -> Mux/6
  Gain/1 -> Mux/3
  Mux/1 -> Scope/1, [F]
  Selector/1 -> [BF_att]
  Gain1/1 -> Scope1/2, Demux1/1
  connections:
  Simulink-PS Converter9/RConn1 -- Mot 5/LConn2
  P4/LConn1 -- Mot 4/RConn1
  Hexa_Simsape/RConn3 -- Mot 3/LConn1
  Hexa_Simsape/RConn6 -- Mot 2/LConn1
  Hexa_Simsape/RConn5 -- Mot 1/LConn1
  Simulink-PS Converter10/RConn1 -- Mot 1/LConn2
  Hexa_Simsape/RConn2 -- Mot 5/LConn1
  Sx4/LConn1 -- Sensor de Rotacion/RConn2
  Hexa_Simsape/RConn4 -- Mot 6/LConn1
  Simulink-PS Converter2/RConn1 -- Mot 4/LConn2
  P1/LConn1 -- Mot 1/RConn1
  P6/LConn1 -- Mot 6/RConn1
  y/LConn1 -- Sensor de Posicion/RConn3
  P2/LConn1 -- Mot 2/RConn1
  Hexa_Simsape/RConn1 -- Mot 4/LConn1
  Sensor de Posicion/RConn4 -- z/LConn1
  Sensor de Posicion/RConn6 -- yp/LConn1
  P3/LConn1 -- Mot 3/RConn1
  Sensor de Posicion/RConn7 -- zp/LConn1
  Sensor de Posicion/RConn1 -- 6-DOF Joint/RConn1 -- Sensor de Rotacion/RConn1 -- 6DOF_Joint/LConn1
  Simulink-PS Converter11/RConn1 -- Mot 2/LConn2
  Sensor de Rotacion/LConn1 -- Infinite Plane2/LConn1 -- Infinite Plane1/LConn1 -- Infinite Plane/LConn1 -- Sensor de Posicion/LConn1 -- MechanismConfiguration2/RConn1 -- 6-DOF Joint/LConn1 -- World2/RConn1 -- Solver Configuration2/RConn1
  Simulink-PS Converter12/RConn1 -- Mot 3/LConn2
  Sensor de Posicion/RConn2 -- x/LConn1
  P5/LConn1 -- Mot 5/RConn1
  Sensor de Posicion/RConn5 -- xp/LConn1
  6DOF_Joint/RConn1 -- Hexa_Simsape/LConn1
  Simulink-PS Converter1/RConn1 -- Mot 6/LConn2
  Sensor de Rotacion/RConn3 -- PS-Simulink Converter3/LConn1
  Sensor de Rotacion/RConn4 -- PS-Simulink Converter4/LConn1
  Sensor de Rotacion/RConn5 -- PS-Simulink Converter5/LConn1

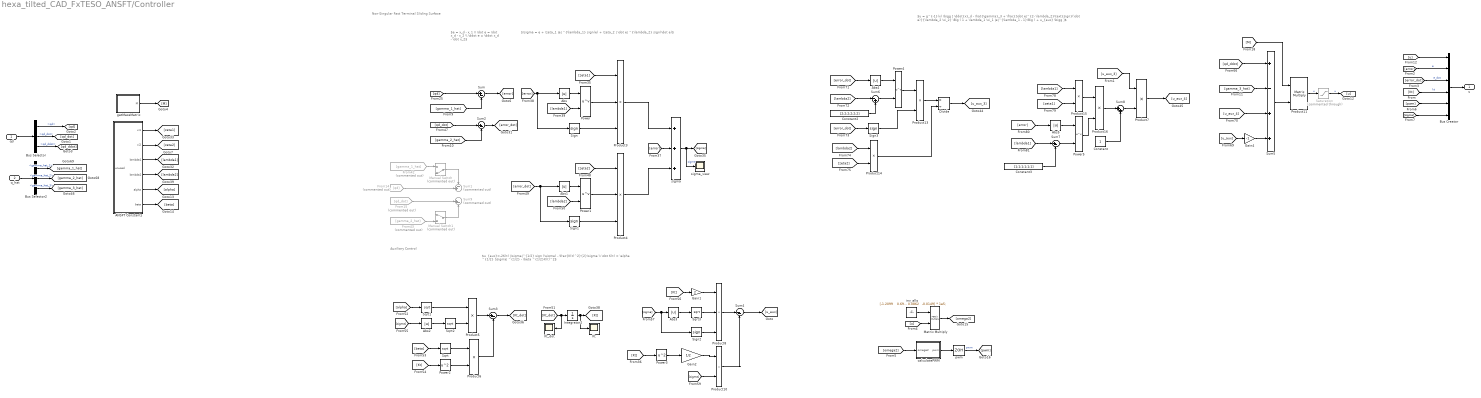
== system hexa_tilted_CAD_FxTESO_ANSFT/Controller ==
  note: $u = g^{-1}(x) \bigg [ \ddot{x}_d - \hat{\gamma}_3 + \frac{|\dot e|^{2- \lambda_2}\text{sign}(\dot e)}{\lambda_2 \xi_2} \Big ( 1 + \lambda_1 \xi_1 |e|^{\lambda_1 - 1}\Big ) + u_{aux} \bigg ]$
  note: Auxiliary Control
  note: Non-Singular Fast Terminal Sliding Surface
  note: $e = x_d - x_1 \\ \dot e = \dot x_d - x_2 \\ \ddot e = \ddot x_d - \dot x_2$
  note: $\sigma = e + \zeta_1 |e| ^{\lambda_1} sign(e) + \zeta_2 | \dot e| ^{\lambda_2} sign(\dot e)$
  note: $u_{aux}=-2K(t) |\sigma|^{1/2} sign (\sigma) - \frac{K(t)^2}{2}\sigma \\ \dot K(t) = \alpha ^{1/2} |\sigma| ^{1/2} - \beta ^{1/2}K(t)^2$
  qd : Inport
  q_hat : Inport  Port=2
  ANSFT Constants : MATLAB Function  TreatAsAtomicUnit=on
  Abs{,1..5} (6 alike) : Abs  SaturateOnIntegerOverflow=off
  Bus Creator : BusCreator  Inputs=6
  Bus Selector : BusSelector  OutputSignals=qd,qd_dot,qd_ddot
  Bus Selector2 : BusSelector  OutputSignals=gamma_hat_1,gamma_hat_2,gamma_hat_3
  Constant : Constant
  Constant2 : Constant  Value=[2;2;2;2;2;2]
  Constant3 : Constant  Value=[1;1;1;1;1;1]
  Divide : Product  Inputs=*/
  From14 : From  Commented=on  GotoTag=qd
  From15 : From  Commented=on  GotoTag=qd_dot
  From42 : From  Commented=on  GotoTag=gamma_1_hat
  From43 : From  Commented=on  GotoTag=gamma_2_hat
  Gain1 : Gain  Gain=2
  Gain2 : Gain  Gain=1/2
  Gain4 : Gain  Gain=-1
  Integrator2 : Integrator  InitialCondition=[0;0;0;0;0;0]
  Kt : Scope
  Kt_dot : Scope
  Manual Switch : ManualSwitch  Commented=on  CurrentSetting=0
  Manual Switch1 : ManualSwitch  Commented=on
  Matrix Multiply : Product  Multiplication=Matrix(*)
  Power{,1,4..5} (4 alike) : Math  Operator=pow
  Power2 : Math  Operator=square
  Power3 : Math  Operator=square
  Product{5..7,10,13..16} (8 alike) : Product
  Product11 : Product  Multiplication=Matrix(*)
  Product3 : Product  Inputs=3
  Product4 : Product  Inputs=3
  Product8 : Product  Inputs=3
  Saturation : Saturate  Commented=through  UpperLimit=[5, 5, 0, 0.5, 0.5, 0.5]'  LowerLimit=[-5, -5, -42, -0.5, -0.5, -0.5]'
  Sign{,1..3} (4 alike) : Signum
  Sqrt{,1..3} (4 alike) : Sqrt
  Sum{,2..3,7} (4 alike) : Sum  Inputs=|+-
  Sum1 : Sum  Commented=on  Inputs=-+|
  Sum4 : Sum  Inputs=|--
  Sum5 : Sum  Inputs=+-++
  Sum6 : Sum  Inputs=|-+
  Sum8 : Sum  Inputs=|++
  Sum9 : Sum  Commented=on  Inputs=|+-
  calculatePWM : MATLAB Function  TreatAsAtomicUnit=on
  getMassMatrix : MATLAB Function  TreatAsAtomicUnit=on
  inv_allo : Constant  Value=|
      | [-1.2099    0.6985    0.2542   -0.0746    0.0431    0.0149;
      |     1.2099    0.6985    0.2542   -0.0746   -0.0431   -0.0149;
      |    -0.0000   -1.3971    0.2542    0.0000   -0.0862    0.0149;
      |    -1.2099    0.6985    0.2542    0.0746   -0.0431   -0.0149;
      |     1.2099    0.6985    0.2542    0.0746    0.0431    0.0149;
      |    -0.0000   -1.3971    0.2542    0.0000    0.0862   -0.0149] * 1e5;
  pwm : ZeroOrderHold  SampleTime=-1
  sigma : Sum  Inputs=+++
  sigma_view : Scope
  u : Outport
  wires:
  Product6/1 -> Sum3/2
  Sign1/1 -> Product4/3
  Sum8/1 -> Product7/2
  Product5/1 -> Sum3/1
  [error_dot] -> Abs4/1
  [u_aux_3] -> Product7/1
  Power5/1 -> Product16/2
  [zeta1] -> Product3/1
  Constant/1 -> Sum8/2
  Product16/1 -> Sum8/1
  Sqrt/1 -> Product6/1
  Product10/1 -> Sum4/2
  Sum6/1 -> Power4/2
  Product15/1 -> Product16/1
  [qd_ddot] -> Sum5/1
  [lambda2] -> Sum6/1
  Sum4/1 -> [u_aux]
  [Kt] -> Power2/1
  Gain1/1 -> Product8/1
  Sum5/1 -> Product11/2
  Sqrt1/1 -> Product5/1
  Constant2/1 -> Sum6/2
  Sign3/1 -> Product13/2
  [lambda1] -> Sum7/1
  [gamma_2_hat] -> Sum2/2
  Power3/1 -> Gain2/1
  Product3/1 -> sigma/1
  [beta] -> Sqrt/1
  Abs4/1 -> Power4/1
  [Kt] -> Gain1/1
  [error_dot] -> Sign1/1, Abs1/1
  Divide/1 -> [u_aux_3]
  [sigma] -> Sign2/1, Abs3/1
  [zeta2] -> Product14/2
  Sum3/1 -> [Kt_dot]
  Product8/1 -> Sum4/1
  [sigma] -> Abs2/1
  Power/1 -> Product3/2
  Product4/1 -> sigma/3
  [u_aux] -> Gain4/1
  Constant3/1 -> Sum7/2
  [error] -> sigma/2
  Abs3/1 -> Sqrt3/1
  [alpha] -> Sqrt1/1
  Sum7/1 -> Power5/2
  Sqrt2/1 -> Product5/2
  Power4/1 -> Product13/1
  [M] -> Product11/1
  sigma/1 -> sigma_view/1, [sigma]  "sigma"
  Sign/1 -> Product3/3
  Abs2/1 -> Sqrt2/1
  [Kt_dot] -> Kt_dot/1, Integrator2/1
  Power1/1 -> Product4/2
  [lambda2] -> Product14/1
  Power2/1 -> Product6/2
  [zeta1] -> Product15/2
  [Kt] -> Power3/1
  [lambda1] -> Product15/1
  [error_dot] -> Sign3/1
  Sqrt3/1 -> Product8/2
  Product13/1 -> Divide/1
  [zeta2] -> Product4/1
  Integrator2/1 -> Kt/1, [Kt]
  [gamma_1_hat] -> Sum/2
  Abs/1 -> Power/1
  [qd] -> Sum/1
  Abs1/1 -> Power1/1
  Sum2/1 -> [error_dot]
  Sum/1 -> [error]
  Gain2/1 -> Product10/1
  Product14/1 -> Divide/2
  [lambda2] -> Power1/2
  [error] -> Abs5/1
  Abs5/1 -> Power5/1
  Product7/1 -> [u_aux_4]
  [sigma] -> Product10/2
  [lambda1] -> Power/2
  Sign2/1 -> Product8/3
  [error] -> Sign/1, Abs/1
  [qd_dot] -> Sum2/1
  Bus Creator/1 -> u/1
  ANSFT Constants/3(lambda1) -> [lambda1]
  ANSFT Constants/1(xi1) -> [zeta1]
  ANSFT Constants/2(xi2) -> [zeta2]
  ANSFT Constants/5(alpha) -> [alpha]
  ANSFT Constants/6(beta) -> [beta]
  ANSFT Constants/4(lambda2) -> [lambda2]
  qd/1 -> Bus Selector/1
  Bus Selector/2 -> [qd_dot]  "<qd_dot>"
  Bus Selector/1 -> [qd]  "<qd>"
  Bus Selector/3 -> [qd_ddot]  "<qd_ddot>"
  Product11/1 -> Saturation/1  "u"
  [error] -> Bus Creator/2  "e"
  [error_dot] -> Bus Creator/3  "e_dot"
  [Kt] -> Bus Creator/4  "kt"
  inv_allo/1 -> Matrix Multiply/1
  [u] -> Matrix Multiply/2
  Matrix Multiply/1 -> [omega2]
  [omega2] -> calculatePWM/1(omega2)
  calculatePWM/1(pwm) -> pwm/1
  pwm/1 -> [pwm]  "pwm"
  [pwm] -> Bus Creator/5
  [sigma] -> Bus Creator/6
  q_hat/1 -> Bus Selector2/1
  Bus Selector2/2 -> [gamma_2_hat]  "<gamma_hat_2>"
  Bus Selector2/3 -> [gamma_3_hat]  "<gamma_hat_3>"
  Bus Selector2/1 -> [gamma_1_hat]  "<gamma_hat_1>"
  [gamma_3_hat] -> Sum5/2
  [u] -> Bus Creator/1
  Saturation/1 -> [u]  "u"
  getMassMatrix/1(M) -> [M]
  From14/1 -> Sum1/2
  From15/1 -> Sum9/1
  Manual Switch1/1 -> Sum9/2
  From43/1 -> Manual Switch1/2
  From42/1 -> Manual Switch/1
  Manual Switch/1 -> Sum1/1
  [u_aux_4] -> Sum5/3
  Gain4/1 -> Sum5/4

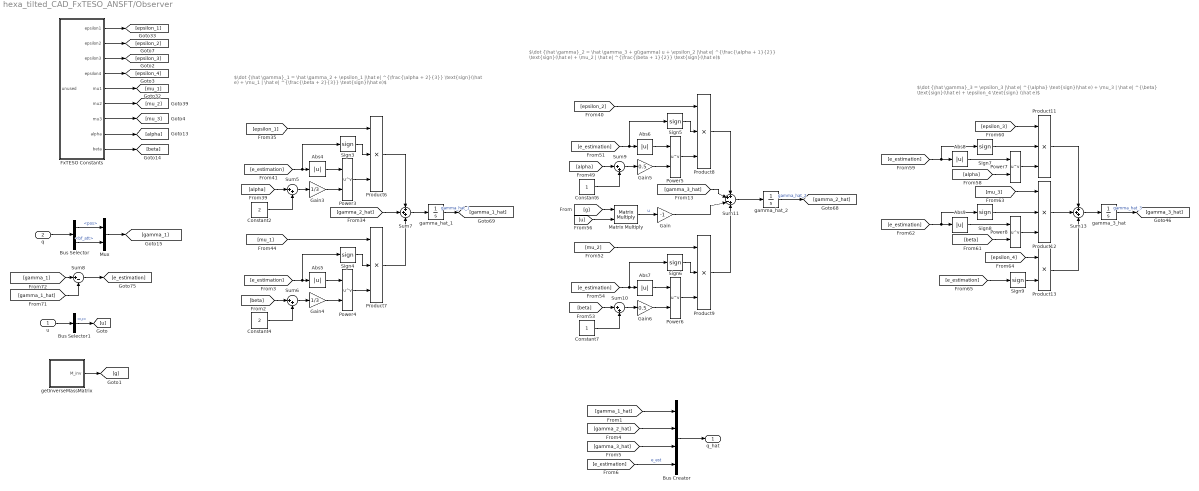
== system hexa_tilted_CAD_FxTESO_ANSFT/Observer ==
  note: $\dot {\hat \gamma}_3 = \epsilon_3 |\hat e| ^{\alpha} \text{sign}(\hat e) + \mu_3 | \hat e| ^{\beta} \text{sign}(\hat e) + \epsilon_4 \text{sign} (\hat e)$
  note: $\dot {\hat \gamma}_1 = \hat \gamma_2 + \epsilon_1 |\hat e| ^{\frac{\alpha + 2}{3}} \text{sign}(\hat e) + \mu_1 | \hat e| ^{\frac{\beta + 2}{3}} \text{sign}(\hat e)$
  note: $\dot {\hat \gamma}_2 = \hat \gamma_3 + g(\gamma) u + \epsilon_2 |\hat e| ^{\frac{\alpha + 1}{2}} \text{sign}(\hat e) + \mu_2 | \hat e| ^{\frac{\beta + 1}{2}} \text{sign}(\hat e)$
  u : Inport
  q : Inport  Port=2
  Abs{4..9} (6 alike) : Abs  SaturateOnIntegerOverflow=off
  Bus Creator : BusCreator  Inputs=4
  Bus Selector : BusSelector  OutputSignals=pos,bf_att
  Bus Selector1 : BusSelector  OutputSignals=u
  Constant2 : Constant  Value=2
  Constant4 : Constant  Value=2
  Constant6 : Constant
  Constant7 : Constant
  FxTESO Constants : MATLAB Function  TreatAsAtomicUnit=on
  Gain : Gain  Gain=-1
  Gain3 : Gain  Gain=1/3
  Gain4 : Gain  Gain=1/3
  Gain5 : Gain  Gain=0.5
  Gain6 : Gain  Gain=0.5
  Matrix Multiply : Product  Multiplication=Matrix(*)
  Mux : Mux  Inputs=2
  Power{3..8} (6 alike) : Math  Operator=pow
  Product{6..9,11..12} (6 alike) : Product  Inputs=3
  Product13 : Product
  Sign{3..9} (7 alike) : Signum
  Sum{5..6,9..10} (4 alike) : Sum  Inputs=|++
  Sum11 : Sum  Inputs=++-+
  Sum13 : Sum  Inputs=+++
  Sum7 : Sum  Inputs=+++
  Sum8 : Sum  Inputs=|+-
  gamma_3_hat : Integrator
  gamma_hat_1 : Integrator
  gamma_hat_2 : Integrator
  getInverseMassMatrix : MATLAB Function  TreatAsAtomicUnit=on
  q_hat : Outport
  wires:
  [gamma_1] -> Sum8/1
  Gain6/1 -> Power6/2
  [alpha] -> Power7/2
  [gamma_3_hat] -> Sum11/2
  Sign7/1 -> Product11/2
  Sum7/1 -> gamma_hat_1/1
  Abs7/1 -> Power6/1
  [gamma_1_hat] -> Sum8/2
  [alpha] -> Sum5/1
  Sum8/1 -> [e_estimation]
  Power4/1 -> Product7/3
  [epsilon_3] -> Product11/1
  Power3/1 -> Product6/3
  Constant2/1 -> Sum5/2
  Abs9/1 -> Power8/1
  Sign5/1 -> Product8/2
  [e_estimation] -> Abs9/1, Sign8/1
  Gain4/1 -> Power4/2
  [e_estimation] -> Sign5/1, Abs6/1
  [mu_3] -> Product12/1
  Power7/1 -> Product11/3
  [beta] -> Power8/2
  Sign8/1 -> Product12/2
  [epsilon_1] -> Product6/1
  Product13/1 -> Sum13/3
  Sign9/1 -> Product13/2
  Sum11/1 -> gamma_hat_2/1
  Sum5/1 -> Gain3/1
  Product7/1 -> Sum7/3
  [e_estimation] -> Sign6/1, Abs7/1
  Abs4/1 -> Power3/1
  Abs8/1 -> Power7/1
  [e_estimation] -> Sign4/1, Abs5/1
  Sum9/1 -> Gain5/1
  [e_estimation] -> Abs8/1, Sign7/1
  Sum13/1 -> gamma_3_hat/1
  [e_estimation] -> Sign3/1, Abs4/1
  Sign6/1 -> Product9/2
  [beta] -> Sum10/1
  Power8/1 -> Product12/3
  Sign3/1 -> Product6/2
  [mu_1] -> Product7/1
  [mu_2] -> Product9/1
  [gamma_2_hat] -> Sum7/2
  [epsilon_4] -> Product13/1
  [beta] -> Sum6/1
  Sum10/1 -> Gain6/1
  Gain3/1 -> Power3/2
  Constant4/1 -> Sum6/2
  gamma_hat_1/1 -> [gamma_1_hat]  "gamma_hat_1"
  [epsilon_2] -> Product8/1
  Abs5/1 -> Power4/1
  Sign4/1 -> Product7/2
  Gain5/1 -> Power5/2
  Product12/1 -> Sum13/2
  gamma_hat_2/1 -> [gamma_2_hat]  "gamma_hat_2"
  Product6/1 -> Sum7/1
  [e_estimation] -> Sign9/1
  Product8/1 -> Sum11/1
  Constant6/1 -> Sum9/2
  [alpha] -> Sum9/1
  Abs6/1 -> Power5/1
  Power6/1 -> Product9/3
  [u] -> Matrix Multiply/2
  Product11/1 -> Sum13/1
  Constant7/1 -> Sum10/2
  gamma_3_hat/1 -> [gamma_3_hat]  "gamma_hat_3"
  Sum6/1 -> Gain4/1
  Power5/1 -> Product8/3
  Matrix Multiply/1 -> Gain/1  "u"
  Product9/1 -> Sum11/4
  FxTESO Constants/5(mu1) -> [mu_1]
  FxTESO Constants/1(epsilon1) -> [epsilon_1]
  FxTESO Constants/2(epsilon2) -> [epsilon_2]
  FxTESO Constants/8(alpha) -> [alpha]
  FxTESO Constants/9(beta) -> [beta]
  FxTESO Constants/6(mu2) -> [mu_2]
  q/1 -> Bus Selector/1
  [g] -> Matrix Multiply/1
  FxTESO Constants/4(epsilon4) -> [epsilon_4]
  FxTESO Constants/3(epsilon3) -> [epsilon_3]
  FxTESO Constants/7(mu3) -> [mu_3]
  u/1 -> Bus Selector1/1
  Bus Selector1/1 -> [u]  "<u>"
  [gamma_1_hat] -> Bus Creator/1
  [gamma_3_hat] -> Bus Creator/3
  [gamma_2_hat] -> Bus Creator/2
  Bus Creator/1 -> q_hat/1
  [e_estimation] -> Bus Creator/4  "e_est"
  Gain/1 -> Sum11/3
  Bus Selector/1 -> Mux/1  "<pos>"
  Bus Selector/2 -> Mux/2  "<bf_att>"
  Mux/1 -> [gamma_1]
  getInverseMassMatrix/1(M_inv) -> [g]
